simulink model "All_Controllers"  (R2019b)
settings: Solver=VariableStepAuto  StartTime=0.0  StopTime=100  RelTol=1e-3
values from neighbouring files (symbols this model uses):
  bike_params = [g h b a lambda m]    [All_ControllersScript.m]
  D_Balancing = 0.0566    [All_ControllersScript.m]
  D_Heading = 0    [All_ControllersScript.m]    (also in Curiving.m)
  D_Lateral = 1    [All_ControllersScript.m]    (also in Curiving.m = 0)
  FinalValue = 1    [All_ControllersScript.m]
  I_Balancing = 1.1908    [All_ControllersScript.m]
  I_Heading = 0    [All_ControllersScript.m]    (also in Curiving.m)
  I_Lateral = 0.1    [All_ControllersScript.m]    (also in Curiving.m = 0.2)
  Init_Angle = 0    [All_ControllersScript.m]
  Init_X = 0    [All_ControllersScript.m]
  Init_Y = 0    [All_ControllersScript.m]
  Init_Yaw = 0    [All_ControllersScript.m]
  lambda = deg2rad(90-24)    [All_ControllersScript.m]
  Noise = 1    [All_ControllersScript.m]
  P_Balancing = 4.8049    [All_ControllersScript.m]
  P_Heading = 0    [All_ControllersScript.m]    (also in Curiving.m = -1)
  P_Lateral = 1    [All_ControllersScript.m]    (also in Curiving.m = 10)
  SimulinkPath = interparc(0:(distanceStep/total_length):1,TestPath(:,1),TestPath(:,2),'linear')    [All_ControllersScript.m]    (also in Curiving.m = PreparedPath{i})
  sys_dicretePID = c2d(steer_sys, Tsm, 'matched')    [All_ControllersScript.m]
  Ts = 0.01    [All_ControllersScript.m]
  TsD = 0.1    [All_ControllersScript.m]
  Tsm = Ts    (= 0.01)    [All_ControllersScript.m]
  v = 10/3.6    (= 2.77777777778)    [All_ControllersScript.m]
undefined symbols (not defined in the file or in its folder): A, B, C, D, data13
libraries: simulink_extras x5, simulink x5
settings Model: Creator=npn13003  LastModifiedBy=hampu
settings DataIOCC: ReturnWorkspaceOutputs=off
settings DebuggingCC: ArithmeticOperatorsInVariantConditions=warning
settings SFSimCC: SimUseLocalCustomCode=off  CustomCodeUndefinedFunction=UseInterfaceOnly
settings RTWCC: RTWUseLocalCustomCode=off

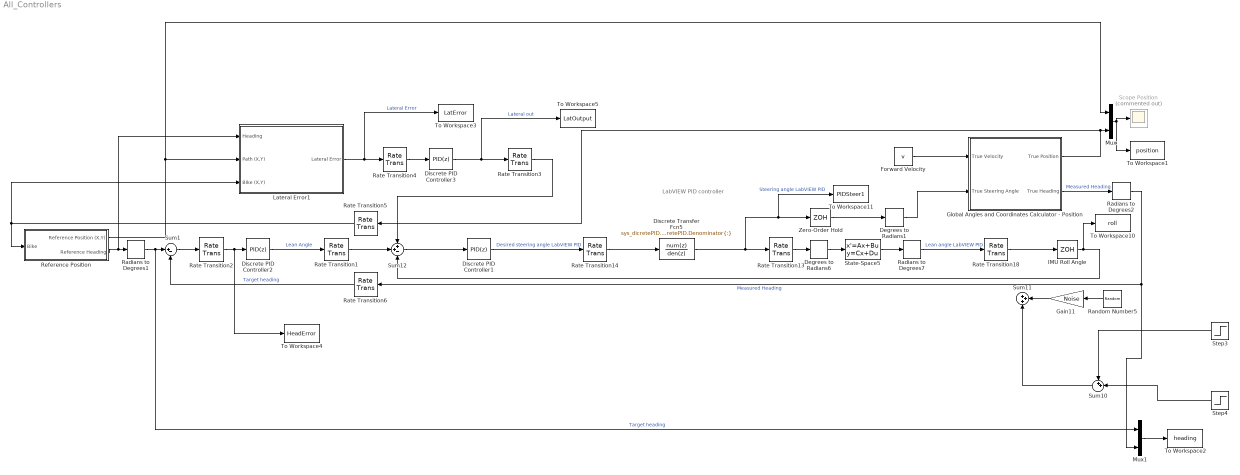
== system All_Controllers ==
  note: LabVIEW PID controller
  Degrees to Radians1 : simulink_extras/Transformations/Degrees to Radians
  Degrees to Radians6 : simulink_extras/Transformations/Degrees to Radians
  Discrete Transfer Fcn5 : DiscreteTransferFcn  Numerator=sys_dicretePID.Numerator{:}  Denominator=sys_dicretePID.Denominator{:}
  Discrete PID Controller1 : simulink/Continuous/PID Controller  Controller=PID  Form=Ideal  TimeDomain=Discrete-time  SampleTime=Ts  IntegratorMethod=Trapezoidal  FilterMethod=Forward Euler  ControllerParametersSource=internal  P=P_Balancing  I=I_Balancing  D=D_Balancing  UseFilter=off  N=100  TunerSelectOption=Transfer Function Based (PID Tuner App)  InitialConditionSource=internal  InitialConditionForIntegrator=0  InitialConditionForFilter=0  DifferentiatorICPrevScaledInput=0  ExternalReset=none  TrackingMode=off  Kt=1  LimitOutput=off  UpperSaturationLimit=inf  LowerSaturationLimit=-inf  LinearizeAsGain=off  AntiWindupMode=none  Kb=1  POutMin=[]  POutMax=[]  IOutMin=[]  IOutMax=[]  DOutMin=[]  DOutMax=[]  NOutMin=[]  NOutMax=[]  SumOutMin=[]  SumOutMax=[]  SaturationOutMin=[]  SaturationOutMax=[]  PParamMin=[]  PParamMax=[]  IParamMin=[]  IParamMax=[]  DParamMin=[]  DParamMax=[]  NParamMin=[]  NParamMax=[]  KbParamMin=[]  KbParamMax=[]  KtParamMin=[]  KtParamMax=[]  KbOutMin=[]  KbOutMax=[]  KtOutMin=[]  KtOutMax=[]  IntegratorOutMin=[]  IntegratorOutMax=[]  FilterOutMin=[]  FilterOutMax=[]  SumI1OutMin=[]  SumI1OutMax=[]  SumI2OutMin=[]  SumI2OutMax=[]  SumI3OutMin=[]  SumI3OutMax=[]  SumI4OutMin=[]  SumI4OutMax=[]  SumDOutMin=[]  SumDOutMax=[]  DifferentiatorOutMin=[]  DifferentiatorOutMax=[]  FilterDiffOutCoefMin=[]  FilterDiffOutCoefMax=[]  ReciprocalOutMin=[]  ReciprocalOutMax=[]  SumDenOutMin=[]  SumDenOutMax=[]  SumNumOutMin=[]  SumNumOutMax=[]  DivideOutMin=[]  DivideOutMax=[]  IntegratorContinuousStateAttributes=''  IntegratorStateMustResolveToSignalObject=off  IntegratorRTWStateStorageClass=Auto  FilterContinuousStateAttributes=''  FilterStateMustResolveToSignalObject=off  FilterRTWStateStorageClass=Auto  ParallelPVariant=Passthrough  IdealPVariant=InternalParameters  IVariant=InternalParameters  DVariant=InternalParameters  IntegratorVariant=Discrete  SatVariant=Disabled  AWVariant=Passthrough  PCopyVariant=Disabled  TRVariant=Disabled  FdbkBlocksVariant=Forward  IdealPFdbkVariant=Disabled  SatFdbkVariant=Disabled  DerivativeFilterVariant=Differentiator  NVariant=Passthrough  NCopyVariant=Disabled_SignalSpec  FilterICVariant=InternalICsDifferentiator  IntegratorICVariant=InternalICs  ExternalResetVariant=Disabled  TRSumVariant=Passthrough  SumFdbkVariant=Disabled  SumVariant=Sum_PID
  Discrete PID Controller2 : simulink/Continuous/PID Controller  Controller=PID  Form=Ideal  TimeDomain=Discrete-time  SampleTime=TsD  IntegratorMethod=Trapezoidal  FilterMethod=Forward Euler  ControllerParametersSource=internal  P=P_Heading  I=I_Heading  D=D_Heading  UseFilter=off  N=100  TunerSelectOption=Transfer Function Based (PID Tuner App)  InitialConditionSource=internal  InitialConditionForIntegrator=0  InitialConditionForFilter=0  DifferentiatorICPrevScaledInput=0  ExternalReset=none  TrackingMode=off  Kt=1  LimitOutput=off  UpperSaturationLimit=inf  LowerSaturationLimit=-inf  LinearizeAsGain=off  AntiWindupMode=none  Kb=1  POutMin=[]  POutMax=[]  IOutMin=[]  IOutMax=[]  DOutMin=[]  DOutMax=[]  NOutMin=[]  NOutMax=[]  SumOutMin=[]  SumOutMax=[]  SaturationOutMin=[]  SaturationOutMax=[]  PParamMin=[]  PParamMax=[]  IParamMin=[]  IParamMax=[]  DParamMin=[]  DParamMax=[]  NParamMin=[]  NParamMax=[]  KbParamMin=[]  KbParamMax=[]  KtParamMin=[]  KtParamMax=[]  KbOutMin=[]  KbOutMax=[]  KtOutMin=[]  KtOutMax=[]  IntegratorOutMin=[]  IntegratorOutMax=[]  FilterOutMin=[]  FilterOutMax=[]  SumI1OutMin=[]  SumI1OutMax=[]  SumI2OutMin=[]  SumI2OutMax=[]  SumI3OutMin=[]  SumI3OutMax=[]  SumI4OutMin=[]  SumI4OutMax=[]  SumDOutMin=[]  SumDOutMax=[]  DifferentiatorOutMin=[]  DifferentiatorOutMax=[]  FilterDiffOutCoefMin=[]  FilterDiffOutCoefMax=[]  ReciprocalOutMin=[]  ReciprocalOutMax=[]  SumDenOutMin=[]  SumDenOutMax=[]  SumNumOutMin=[]  SumNumOutMax=[]  DivideOutMin=[]  DivideOutMax=[]  IntegratorContinuousStateAttributes=''  IntegratorStateMustResolveToSignalObject=off  IntegratorRTWStateStorageClass=Auto  FilterContinuousStateAttributes=''  FilterStateMustResolveToSignalObject=off  FilterRTWStateStorageClass=Auto  ParallelPVariant=Passthrough  IdealPVariant=InternalParameters  IVariant=InternalParameters  DVariant=InternalParameters  IntegratorVariant=Discrete  SatVariant=Disabled  AWVariant=Passthrough  PCopyVariant=Disabled  TRVariant=Disabled  FdbkBlocksVariant=Forward  IdealPFdbkVariant=Disabled  SatFdbkVariant=Disabled  DerivativeFilterVariant=Differentiator  NVariant=Passthrough  NCopyVariant=Disabled_SignalSpec  FilterICVariant=InternalICsDifferentiator  IntegratorICVariant=InternalICs  ExternalResetVariant=Disabled  TRSumVariant=Passthrough  SumFdbkVariant=Disabled  SumVariant=Sum_PID
  Discrete PID Controller3 : simulink/Continuous/PID Controller  Controller=PID  Form=Ideal  TimeDomain=Discrete-time  SampleTime=TsD  IntegratorMethod=Trapezoidal  FilterMethod=Forward Euler  ControllerParametersSource=internal  P=-P_Lateral  I=I_Lateral  D=D_Lateral  UseFilter=off  N=100  TunerSelectOption=Transfer Function Based (PID Tuner App)  InitialConditionSource=internal  InitialConditionForIntegrator=0  InitialConditionForFilter=0  DifferentiatorICPrevScaledInput=0  ExternalReset=none  TrackingMode=off  Kt=1  LimitOutput=off  UpperSaturationLimit=inf  LowerSaturationLimit=-inf  LinearizeAsGain=off  AntiWindupMode=none  Kb=1  POutMin=[]  POutMax=[]  IOutMin=[]  IOutMax=[]  DOutMin=[]  DOutMax=[]  NOutMin=[]  NOutMax=[]  SumOutMin=[]  SumOutMax=[]  SaturationOutMin=[]  SaturationOutMax=[]  PParamMin=[]  PParamMax=[]  IParamMin=[]  IParamMax=[]  DParamMin=[]  DParamMax=[]  NParamMin=[]  NParamMax=[]  KbParamMin=[]  KbParamMax=[]  KtParamMin=[]  KtParamMax=[]  KbOutMin=[]  KbOutMax=[]  KtOutMin=[]  KtOutMax=[]  IntegratorOutMin=[]  IntegratorOutMax=[]  FilterOutMin=[]  FilterOutMax=[]  SumI1OutMin=[]  SumI1OutMax=[]  SumI2OutMin=[]  SumI2OutMax=[]  SumI3OutMin=[]  SumI3OutMax=[]  SumI4OutMin=[]  SumI4OutMax=[]  SumDOutMin=[]  SumDOutMax=[]  DifferentiatorOutMin=[]  DifferentiatorOutMax=[]  FilterDiffOutCoefMin=[]  FilterDiffOutCoefMax=[]  ReciprocalOutMin=[]  ReciprocalOutMax=[]  SumDenOutMin=[]  SumDenOutMax=[]  SumNumOutMin=[]  SumNumOutMax=[]  DivideOutMin=[]  DivideOutMax=[]  IntegratorContinuousStateAttributes=''  IntegratorStateMustResolveToSignalObject=off  IntegratorRTWStateStorageClass=Auto  FilterContinuousStateAttributes=''  FilterStateMustResolveToSignalObject=off  FilterRTWStateStorageClass=Auto  ParallelPVariant=Passthrough  IdealPVariant=InternalParameters  IVariant=InternalParameters  DVariant=InternalParameters  IntegratorVariant=Discrete  SatVariant=Disabled  AWVariant=Passthrough  PCopyVariant=Disabled  TRVariant=Disabled  FdbkBlocksVariant=Forward  IdealPFdbkVariant=Disabled  SatFdbkVariant=Disabled  DerivativeFilterVariant=Differentiator  NVariant=Passthrough  NCopyVariant=Disabled_SignalSpec  FilterICVariant=InternalICsDifferentiator  IntegratorICVariant=InternalICs  ExternalResetVariant=Disabled  TRSumVariant=Passthrough  SumFdbkVariant=Disabled  SumVariant=Sum_PID
  Forward Velocity : Constant  Value=v
  Gain11 : Gain  Gain=Noise
  Global Angles and Coordinates Calculator - Position : Subsystem  SystemSampleTime=Ts
  IMU Roll Angle : ZeroOrderHold  SampleTime=Ts
  Lateral Error1 : Subsystem  SystemSampleTime=Ts
  Mux : Mux  Inputs=2
  Mux1 : Mux  Inputs=2
  Radians to Degrees1 : simulink_extras/Transformations/Radians to Degrees
  Radians to Degrees2 : simulink_extras/Transformations/Radians to Degrees
  Radians to Degrees7 : simulink_extras/Transformations/Radians to Degrees
  Random Number5 : RandomNumber  Variance=0.0001  SampleTime=Ts
  Rate Transition1 : RateTransition  OutPortSampleTime=Ts
  Rate Transition13 : RateTransition  OutPortSampleTime=0
  Rate Transition14 : RateTransition  OutPortSampleTime=Tsm
  Rate Transition18 : RateTransition  OutPortSampleTime=Ts
  Rate Transition{2,4..6} (4 alike) : RateTransition  OutPortSampleTime=TsD
  Rate Transition3 : RateTransition  OutPortSampleTime=Ts
  Reference Position : Subsystem
  Scope Position : Scope  Commented=on
  State-Space5 : StateSpace  A=A  B=B  C=C  D=D  InitialCondition=[deg2rad(Init_Angle/C(1,1)) 0]
  Step3 : Step  Time=1.25  After=-FinalValue  SampleTime=Ts  VectorParams1D=off
  Step4 : Step  After=FinalValue  SampleTime=Ts  VectorParams1D=off
  Sum1 : Sum  Inputs=|+-
  Sum10 : Sum  Inputs=++|
  Sum11 : Sum  Inputs=+++
  Sum12 : Sum  Inputs=++-
  To Workspace1 : ToWorkspace  VariableName=position  SaveFormat=Timeseries  SampleTime=-1
  To Workspace10 : ToWorkspace  VariableName=roll  SaveFormat=Timeseries  SampleTime=-1
  To Workspace11 : ToWorkspace  VariableName=PIDSteer1  SaveFormat=Timeseries  SampleTime=-1
  To Workspace2 : ToWorkspace  VariableName=heading  SaveFormat=Timeseries  SampleTime=-1
  To Workspace3 : ToWorkspace  VariableName=LatError  SaveFormat=Timeseries  SampleTime=-1
  To Workspace4 : ToWorkspace  VariableName=HeadError  SaveFormat=Timeseries  SampleTime=-1
  To Workspace5 : ToWorkspace  VariableName=LatOutput  SaveFormat=Timeseries  SampleTime=-1
  Zero-Order Hold : ZeroOrderHold  SampleTime=Tsm
  wires:
  Step3/1 -> Sum10/1
  Step4/1 -> Sum10/2
  Rate Transition18/1 -> IMU Roll Angle/1
  Degrees to Radians6/1 -> State-Space5/1
  Radians to Degrees7/1 -> Rate Transition18/1  "Lean angle LabVIEW PID"
  Rate Transition14/1 -> Discrete Transfer Fcn5/1
  Rate Transition13/1 -> Degrees to Radians6/1
  State-Space5/1 -> Radians to Degrees7/1
  Random Number5/1 -> Gain11/1
  Discrete Transfer Fcn5/1 -> Zero-Order Hold/1, To Workspace11/1, Rate Transition13/1  "Steering angle LabVIEW PID"
  Discrete PID Controller1/1 -> Rate Transition14/1  "Desired steering angle LabVIEW PID"
  Gain11/1 -> Sum11/2
  Sum10/1 -> Sum11/3
  Sum12/1 -> Discrete PID Controller1/1
  Discrete PID Controller2/1 -> Rate Transition1/1  "Lean Angle"
  Sum1/1 -> Rate Transition2/1
  Reference Position/2(Reference Heading) -> Lateral Error1/1(Heading), Radians to Degrees1/1
  Rate Transition2/1 -> To Workspace4/1, Discrete PID Controller2/1
  IMU Roll Angle/1 -> To Workspace10/1, Sum12/3
  Mux/1 -> To Workspace1/1, Scope Position/1
  Zero-Order Hold/1 -> Degrees to Radians1/1
  Forward Velocity/1 -> Global Angles and Coordinates Calculator - Position/1(True Velocity)
  Degrees to Radians1/1 -> Global Angles and Coordinates Calculator - Position/2(True Steering Angle)
  Radians to Degrees1/1 -> Mux1/1, Sum1/1  "Target heading"
  Global Angles and Coordinates Calculator - Position/2(True Heading) -> Radians to Degrees2/1  "Measured Heading"
  Rate Transition4/1 -> Discrete PID Controller3/1
  Rate Transition3/1 -> Sum12/1
  Discrete PID Controller3/1 -> To Workspace5/1, Rate Transition3/1  "Lateral out"
  Reference Position/1(Reference Position (X,Y)) -> Mux/1, Lateral Error1/2(Path (X,Y))
  Rate Transition1/1 -> Sum12/2
  Mux1/1 -> To Workspace2/1
  Radians to Degrees2/1 -> Rate Transition6/1, Mux1/2  "Measured Heading"
  Global Angles and Coordinates Calculator - Position/1(True Position) -> Rate Transition5/1, Mux/2
  Rate Transition5/1 -> Lateral Error1/3(BIke (X,Y)), Reference Position/1(Bike)
  Lateral Error1/1(Lateral Error) -> To Workspace3/1, Rate Transition4/1  "Lateral Error"
  Rate Transition6/1 -> Sum1/2  "Target heading"

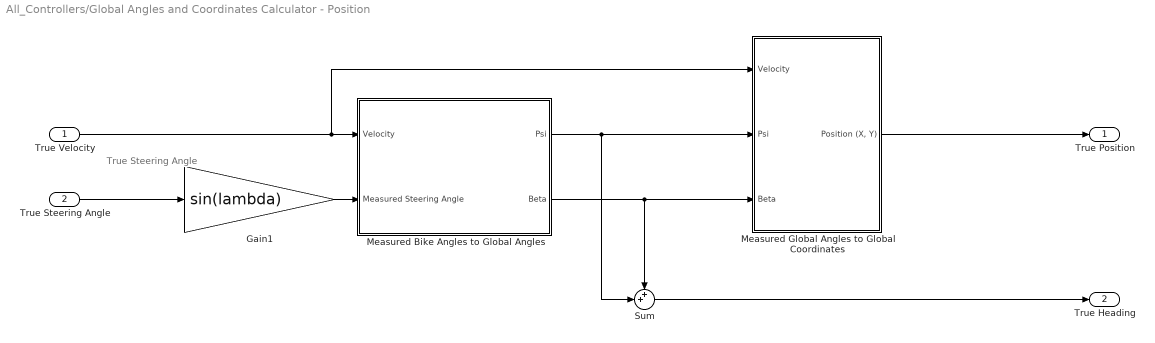
== system All_Controllers/Global Angles and Coordinates Calculator - Position ==
  note: True Steering
      | Angle
  True Velocity : Inport
  True Steering Angle : Inport  Port=2
  Gain1 : Gain  Gain=sin(lambda)
  Measured Bike Angles to Global Angles : Subsystem
  Measured Global Angles to Global Coordinates : Subsystem
  Sum : Sum  Inputs=++|
  True Position : Outport  VectorParamsAs1DForOutWhenUnconnected=off
  True Heading : Outport  Port=2  VectorParamsAs1DForOutWhenUnconnected=off
  wires:
  Measured Bike Angles to Global Angles/1(Psi) -> Sum/2, Measured Global Angles to Global Coordinates/2(Psi)
  Gain1/1 -> Measured Bike Angles to Global Angles/2(Measured Steering Angle)
  Sum/1 -> True Heading/1
  Measured Bike Angles to Global Angles/2(Beta) -> Sum/1, Measured Global Angles to Global Coordinates/3(Beta)
  Measured Global Angles to Global Coordinates/1("Position (X, Y)") -> True Position/1
  True Velocity/1 -> Measured Global Angles to Global Coordinates/1(Velocity), Measured Bike Angles to Global Angles/1(Velocity)
  True Steering Angle/1 -> Gain1/1

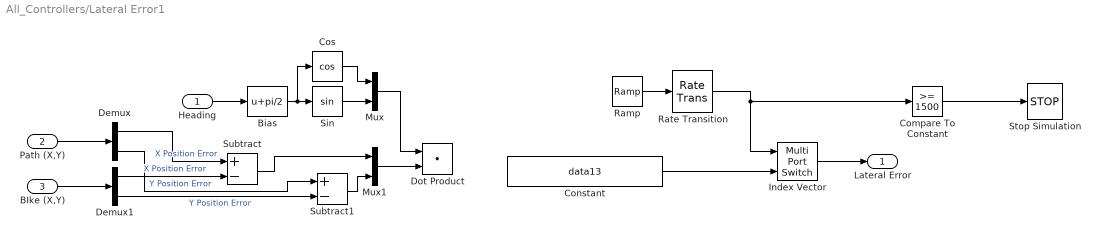
== system All_Controllers/Lateral Error1 ==
  Heading : Inport
  Path (X,Y) : Inport  Port=2
  BIke (X,Y) : Inport  Port=3
  Bias : Bias  Bias=pi/2
  Compare To Constant : simulink/Logic and Bit Operations/Compare To Constant  relop=>=  const=1500  OutDataTypeStr=boolean
  Constant : Constant  Value=data13  VectorParams1D=off  SampleTime=Ts
  Cos : Trigonometry  Operator=cos
  Demux : Demux  Outputs=2
  Demux1 : Demux  Outputs=2
  Dot Product : DotProduct  InputSameDT=on  OutDataTypeStr=Inherit: Inherit via internal rule
  Index Vector : MultiPortSwitch  Inputs=1
  Mux : Mux  Inputs=2
  Mux1 : Mux  Inputs=2
  Ramp : simulink/Sources/Ramp  slope=100  start=0  InitialOutput=1
  Rate Transition : RateTransition  Integrity=off  OutPortSampleTime=Ts
  Sin : Trigonometry
  Stop Simulation : Stop
  Subtract : Sum  Inputs=+-
  Subtract1 : Sum  Inputs=+-
  Lateral Error : Outport  VectorParamsAs1DForOutWhenUnconnected=off
  wires:
  Path (X,Y)/1 -> Demux/1
  BIke (X,Y)/1 -> Demux1/1
  Demux1/1 -> Subtract/2  "X Position Error"
  Demux/1 -> Subtract/1  "X Position Error"
  Demux1/2 -> Subtract1/2  "Y Position Error"
  Demux/2 -> Subtract1/1  "Y Position Error"
  Heading/1 -> Bias/1
  Bias/1 -> Cos/1, Sin/1
  Cos/1 -> Mux/1
  Sin/1 -> Mux/2
  Subtract1/1 -> Mux1/2
  Subtract/1 -> Mux1/1
  Mux/1 -> Dot Product/1
  Mux1/1 -> Dot Product/2
  Constant/1 -> Index Vector/2
  Index Vector/1 -> Lateral Error/1
  Ramp/1 -> Rate Transition/1
  Rate Transition/1 -> Compare To Constant/1, Index Vector/1
  Compare To Constant/1 -> Stop Simulation/1

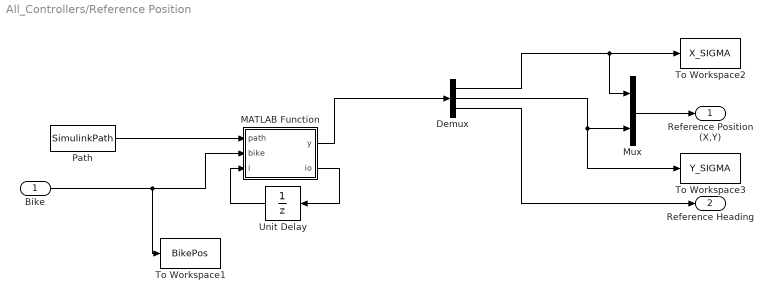
== system All_Controllers/Reference Position ==
  Bike : Inport
  Demux : Demux  Outputs=3
  MATLAB Function : MATLAB Function  TreatAsAtomicUnit=on
  Mux : Mux  Inputs=2
  Path : Constant  Value=SimulinkPath  SampleTime=TsD
  To Workspace1 : ToWorkspace  VariableName=BikePos  SaveFormat=Timeseries  SampleTime=TsD
  To Workspace2 : ToWorkspace  VariableName=X_SIGMA  SaveFormat=Timeseries  SampleTime=TsD
  To Workspace3 : ToWorkspace  VariableName=Y_SIGMA  SaveFormat=Timeseries  SampleTime=TsD
  Unit Delay : UnitDelay  InitialCondition=1  SampleTime=TsD  HasFrameUpgradeWarning=on
  Reference Position (X,Y) : Outport  VectorParamsAs1DForOutWhenUnconnected=off
  Reference Heading : Outport  Port=2  VectorParamsAs1DForOutWhenUnconnected=off
  wires:
  Mux/1 -> Reference Position (X,Y)/1
  Demux/2 -> To Workspace3/1, Mux/2
  Demux/3 -> Reference Heading/1
  Bike/1 -> To Workspace1/1, MATLAB Function/2(bike)
  Path/1 -> MATLAB Function/1(path)
  MATLAB Function/2(io) -> Unit Delay/1
  Unit Delay/1 -> MATLAB Function/3(i)
  Demux/1 -> To Workspace2/1, Mux/1
  MATLAB Function/1(y) -> Demux/1

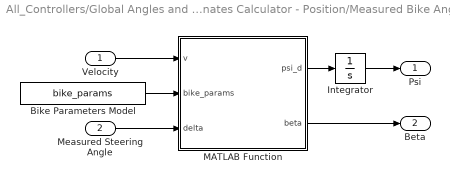
== system All_Controllers/Global Angles and Coordinates Calculator - Position/Measured Bike Angles to Global Angles ==
  Velocity : Inport
  Measured Steering Angle : Inport  Port=2
  " Bike Parameters Model " : Constant  Value=bike_params
  Integrator : Integrator  InitialCondition=deg2rad(Init_Yaw)
  MATLAB Function : MATLAB Function  TreatAsAtomicUnit=on
  Psi : Outport  VectorParamsAs1DForOutWhenUnconnected=off
  Beta : Outport  Port=2  VectorParamsAs1DForOutWhenUnconnected=off
  wires:
  MATLAB Function/2(beta) -> Beta/1
  MATLAB Function/1(psi_d) -> Integrator/1
  Integrator/1 -> Psi/1
  " Bike Parameters Model "/1 -> MATLAB Function/2(bike_params)
  Measured Steering Angle/1 -> MATLAB Function/3(delta)
  Velocity/1 -> MATLAB Function/1(v)

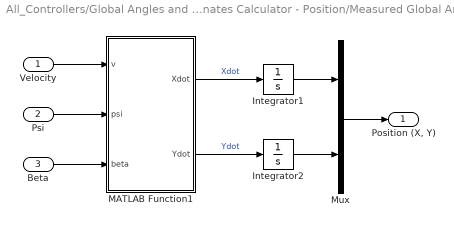
== system All_Controllers/Global Angles and Coordinates Calculator - Position/Measured Global Angles to Global Coordinates ==
  Velocity : Inport
  Psi : Inport  Port=2
  Beta : Inport  Port=3
  Integrator1 : Integrator  InitialCondition=Init_X
  Integrator2 : Integrator  InitialCondition=Init_Y
  MATLAB Function1 : MATLAB Function  TreatAsAtomicUnit=on
  Mux : Mux  Inputs=2
  "Position (X, Y)" : Outport  VectorParamsAs1DForOutWhenUnconnected=off
  wires:
  MATLAB Function1/2(Ydot) -> Integrator2/1  "Ydot"
  MATLAB Function1/1(Xdot) -> Integrator1/1  "Xdot"
  Psi/1 -> MATLAB Function1/2(psi)
  Beta/1 -> MATLAB Function1/3(beta)
  Velocity/1 -> MATLAB Function1/1(v)
  Integrator2/1 -> Mux/2
  Integrator1/1 -> Mux/1
  Mux/1 -> "Position (X, Y)"/1

== matlab function All_Controllers/Reference Position/MATLAB Function ==
  data: path input; bike input; y output; i input; io output
function [y,io] = fcn(path,bike,i)
    j = i;
    usnit = 1;
    y = path(j,:);
    io = 1;
    while(j < length(path) && usnit >= 0)
        n = [cos(path(j,3)) sin(path(j,3))];
        usnit = dot([bike(1)-path(j,1), bike(2)-path(j,2)],n); 
        if(usnit >= 0)
           y =  path(j,:);
           io = j;
        end
        j = j+1;
    end
end

== matlab function All_Controllers/Global Angles and Coordinates Calculator - Position/Measured Bike Angles to Global Angles/MATLAB Function ==
  data: v input; bike_params input; delta input; psi_d output; beta output
function [psi_d, beta]  = fcn(v, bike_params, delta)

b = bike_params(3);
a = bike_params(4);

beta = atan((a / (b)) * tan(delta));
psi_d = (v / a) * sin(beta);

== matlab function All_Controllers/Global Angles and Coordinates Calculator - Position/Measured Global Angles to Global Coordinates/MATLAB Function1 ==
  data: v input; psi input; Xdot output; beta input; Ydot output
function [Xdot, Ydot]  = fcn(v, psi, beta)

Xdot = v * cos(psi + beta);
Ydot = v * sin(psi + beta);
